simulink model "StateFlow_1"  (R2017b)
settings: Solver=FixedStepDiscrete  StartTime=0.0  StopTime=20000  FixedStep=1  RelTol=1e-3
settings Model: Creator=Administrator  LastModifiedBy=Administrator
settings OptimizationCC: DefaultParameterBehavior=Inlined  UseDivisionForNetSlopeComputation=on  UseFloatMulNetSlope=on  InlineInvariantSignals=on  PassReuseOutputArgsAs=Individual arguments  ZeroExternalMemoryAtStartup=off  ZeroInternalMemoryAtStartup=off  NoFixptDivByZeroProtection=on  EfficientFloat2IntCast=on  LifeSpan=1
settings DebuggingCC: ParameterOverflowMsg=none  ParameterTunabilityLossMsg=error  SFUnexpectedBacktrackingDiag=warning  SFNoUnconditionalDefaultTransitionDiag=warning  SFOutputUsedAsStateInMooreChartDiag=warning
settings HardwareCC: ProdBitPerChar=16  ProdBitPerInt=16  ProdBitPerPointer=32  ProdBitPerSizeT=32  ProdBitPerPtrDiffT=32  ProdLargestAtomicInteger=Integer  ProdLargestAtomicFloat=None  ProdWordSize=16  ProdLongLongMode=on  ProdHWDeviceType=Texas Instruments->C2000
settings SFSimCC: MATLABDynamicMemAlloc=off
settings RTWCC: SystemTargetFile=ert.tlc  TemplateMakefile=ert_default_tmf  GenerateReport=on  IncludeHyperlinkInReport=on  LaunchReport=on  GenerateTraceInfo=on  GenerateTraceReport=on  GenerateTraceReportSl=on  GenerateTraceReportSf=on  GenerateTraceReportEml=on  GenerateCodeMetricsReport=on
settings CodeAppCC: ForceParamTrailComments=on  IgnoreCustomStorageClasses=off  OperatorAnnotations=on  SimulinkDataObjDesc=on  SFDataObjDesc=on  CustomSymbolStrGlobalVar=rt$N$M  CustomSymbolStrType=$N$M  CustomSymbolStrFcn=$N$M$F  CustomSymbolStrMacro=$N$M  InsertBlockDesc=on
settings ERTTargetCC: TargetLangStandard=C99 (ISO)  GenerateSampleERTMain=on  IncludeMdlTerminateFcn=off  CombineSignalStateStructs=on  SupportAbsoluteTime=off  SupportComplex=off  SupportNonInlinedSFcns=on  InlinedParameterPlacement=NonHierarchical  ERTCustomFileTemplate=example_file_process.tlc  ERTFilePackagingFormat=CompactWithDataFile
settings ConfigComp: DVMaxProcessTime=1000  DVTestSuiteOptimization=CombinedObjectives (Nonlinear Extended)  DVDetectFloatOverflow=off

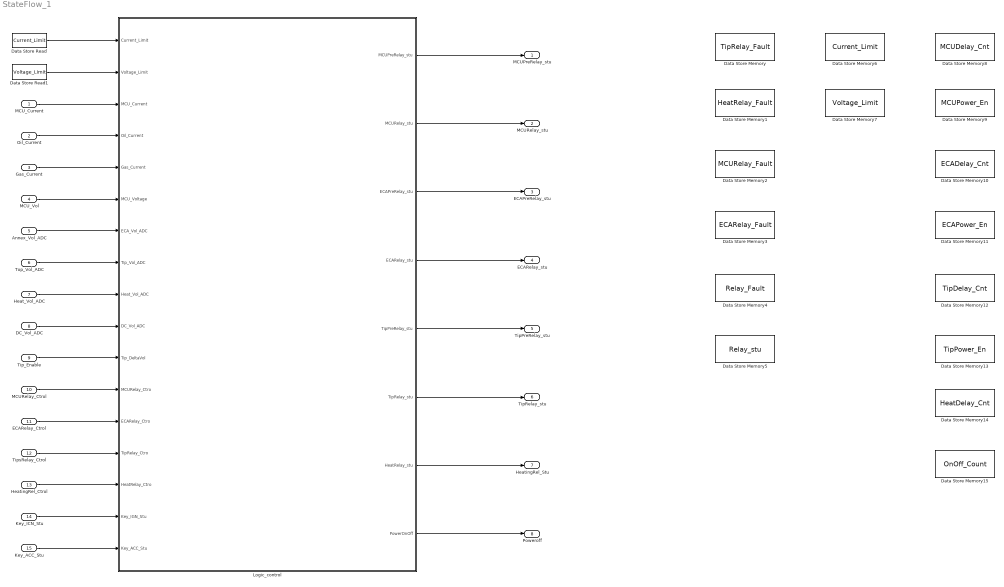
== system StateFlow_1 ==
  MCU_Current : Inport
  Oil_Current : Inport  Port=2
  Gas_Current : Inport  Port=3
  MCU_Vol : Inport  Port=4
  Annex_Vol_ADC : Inport  Port=5
  Top_Vol_ADC : Inport  Port=6
  Heat_Vol_ADC : Inport  Port=7
  DC_Vol_ADC : Inport  Port=8
  Tip_Enable : Inport  Port=9
  MCURelay_Ctrol : Inport  Port=10
  ECARelay_Ctrol : Inport  Port=11
  TipsRelay_Ctrol : Inport  Port=12
  HeatingRel_Ctrol : Inport  Port=13
  Key_ICN_Stu : Inport  Port=14
  Key_ACC_Stu : Inport  Port=15
  Data Store Memory : DataStoreMemory  DataStoreName=TipRelay_Fault  ReadBeforeWriteMsg=warning  WriteAfterWriteMsg=warning  WriteAfterReadMsg=warning  ShowAdditionalParam=off  OutDataTypeStr=uint8
  Data Store Memory1 : DataStoreMemory  DataStoreName=HeatRelay_Fault  ReadBeforeWriteMsg=warning  WriteAfterWriteMsg=warning  WriteAfterReadMsg=warning  ShowAdditionalParam=off  OutDataTypeStr=uint8
  Data Store Memory10 : DataStoreMemory  DataStoreName=ECADelay_Cnt  ReadBeforeWriteMsg=warning  WriteAfterWriteMsg=warning  WriteAfterReadMsg=warning  ShowAdditionalParam=off  OutDataTypeStr=uint16
  Data Store Memory11 : DataStoreMemory  DataStoreName=ECAPower_En  ReadBeforeWriteMsg=warning  WriteAfterWriteMsg=warning  WriteAfterReadMsg=warning  ShowAdditionalParam=off  OutDataTypeStr=uint16
  Data Store Memory12 : DataStoreMemory  DataStoreName=TipDelay_Cnt  ReadBeforeWriteMsg=warning  WriteAfterWriteMsg=warning  WriteAfterReadMsg=warning  ShowAdditionalParam=off  OutDataTypeStr=uint16
  Data Store Memory13 : DataStoreMemory  DataStoreName=TipPower_En  ReadBeforeWriteMsg=warning  WriteAfterWriteMsg=warning  WriteAfterReadMsg=warning  ShowAdditionalParam=off  OutDataTypeStr=uint16
  Data Store Memory14 : DataStoreMemory  DataStoreName=HeatDelay_Cnt  ReadBeforeWriteMsg=warning  WriteAfterWriteMsg=warning  WriteAfterReadMsg=warning  ShowAdditionalParam=off  OutDataTypeStr=uint16
  Data Store Memory15 : DataStoreMemory  DataStoreName=OnOff_Count  ReadBeforeWriteMsg=warning  WriteAfterWriteMsg=warning  WriteAfterReadMsg=warning  ShowAdditionalParam=off  OutDataTypeStr=uint16
  Data Store Memory2 : DataStoreMemory  DataStoreName=MCURelay_Fault  ReadBeforeWriteMsg=warning  WriteAfterWriteMsg=warning  WriteAfterReadMsg=warning  ShowAdditionalParam=off  OutDataTypeStr=uint8
  Data Store Memory3 : DataStoreMemory  DataStoreName=ECARelay_Fault  ReadBeforeWriteMsg=warning  WriteAfterWriteMsg=warning  WriteAfterReadMsg=warning  ShowAdditionalParam=off  OutDataTypeStr=uint8
  Data Store Memory4 : DataStoreMemory  DataStoreName=Relay_Fault  ReadBeforeWriteMsg=warning  WriteAfterWriteMsg=warning  WriteAfterReadMsg=warning  ShowAdditionalParam=off  OutDataTypeStr=uint8
  Data Store Memory5 : DataStoreMemory  DataStoreName=Relay_stu  ReadBeforeWriteMsg=warning  WriteAfterWriteMsg=warning  WriteAfterReadMsg=warning  ShowAdditionalParam=off  OutDataTypeStr=uint8
  Data Store Memory6 : DataStoreMemory  DataStoreName=Current_Limit  ReadBeforeWriteMsg=warning  WriteAfterWriteMsg=warning  WriteAfterReadMsg=warning  InitialValue=15  ShowAdditionalParam=off  OutDataTypeStr=uint16
  Data Store Memory7 : DataStoreMemory  DataStoreName=Voltage_Limit  ReadBeforeWriteMsg=warning  WriteAfterWriteMsg=warning  WriteAfterReadMsg=warning  InitialValue=40  ShowAdditionalParam=off  OutDataTypeStr=uint16
  Data Store Memory8 : DataStoreMemory  DataStoreName=MCUDelay_Cnt  ReadBeforeWriteMsg=warning  WriteAfterWriteMsg=warning  WriteAfterReadMsg=warning  ShowAdditionalParam=off  OutDataTypeStr=uint16
  Data Store Memory9 : DataStoreMemory  DataStoreName=MCUPower_En  ReadBeforeWriteMsg=warning  WriteAfterWriteMsg=warning  WriteAfterReadMsg=warning  ShowAdditionalParam=off  OutDataTypeStr=uint16
  Data Store Read : DataStoreRead  DataStoreName=Current_Limit
  Data Store Read1 : DataStoreRead  DataStoreName=Voltage_Limit
  Logic_control : Subsystem  TreatAsAtomicUnit=on
  MCUPreRelay_stu : Outport
  MCURelay_stu : Outport  Port=2
  ECAPreRelay_stu : Outport  Port=3
  ECARelay_stu : Outport  Port=4
  TipPreRelay_stu : Outport  Port=5
  TipRelay_stu : Outport  Port=6
  HeatingRel_Stu : Outport  Port=7
  Poweroff : Outport  Port=8
  wires:
  Data Store Read/1 -> Logic_control/1(Current_Limit)
  Data Store Read1/1 -> Logic_control/2(Voltage_Limit)
  MCU_Current/1 -> Logic_control/3(MCU_Current)
  Oil_Current/1 -> Logic_control/4(Oil_Current)
  Gas_Current/1 -> Logic_control/5(Gas_Current)
  MCU_Vol/1 -> Logic_control/6(MCU_Voltage)
  MCURelay_Ctrol/1 -> Logic_control/12(MCURelay_Ctro)
  ECARelay_Ctrol/1 -> Logic_control/13(ECARelay_Ctro)
  TipsRelay_Ctrol/1 -> Logic_control/14(TipRelay_Ctro)
  HeatingRel_Ctrol/1 -> Logic_control/15(HeatRelay_Ctro)
  Key_ICN_Stu/1 -> Logic_control/16(Key_IGN_Stu)
  Key_ACC_Stu/1 -> Logic_control/17(Key_ACC_Stu)
  Logic_control/1(MCUPreRelay_stu) -> MCUPreRelay_stu/1
  Logic_control/2(MCURelay_stu) -> MCURelay_stu/1
  Logic_control/3(ECAPreRelay_stu) -> ECAPreRelay_stu/1
  Logic_control/4(ECARelay_stu) -> ECARelay_stu/1
  Logic_control/5(TipPreRelay_stu) -> TipPreRelay_stu/1
  Logic_control/6(TipRelay_stu) -> TipRelay_stu/1
  Logic_control/7(HeatRelay_stu) -> HeatingRel_Stu/1
  Logic_control/8(PowerOnOff) -> Poweroff/1
  Annex_Vol_ADC/1 -> Logic_control/7(ECA_Vol_ADC)
  Top_Vol_ADC/1 -> Logic_control/8(Tip_Vol_ADC)
  Heat_Vol_ADC/1 -> Logic_control/9(Heat_Vol_ADC)
  DC_Vol_ADC/1 -> Logic_control/10(DC_Vol_ADC)
  Tip_Enable/1 -> Logic_control/11(Tip_DeltaVol)

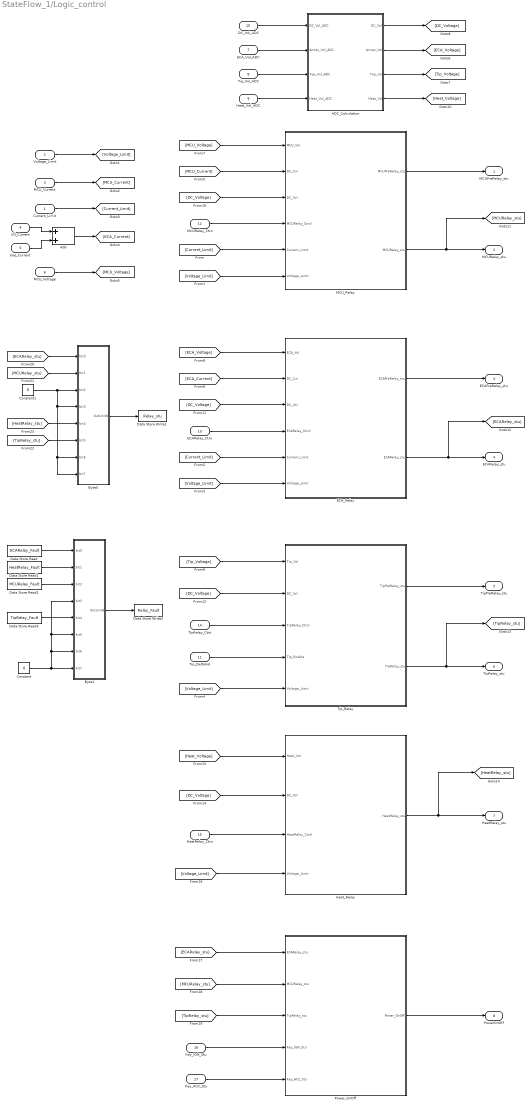
== system StateFlow_1/Logic_control ==
  Current_Limit : Inport
  Voltage_Limit : Inport  Port=2
  MCU_Current : Inport  Port=3
  Oil_Current : Inport  Port=4
  Gas_Current : Inport  Port=5
  MCU_Voltage : Inport  Port=6
  ECA_Vol_ADC : Inport  Port=7
  Tip_Vol_ADC : Inport  Port=8
  Heat_Vol_ADC : Inport  Port=9
  DC_Vol_ADC : Inport  Port=10
  Tip_DeltaVol : Inport  Port=11
  MCURelay_Ctro : Inport  Port=12
  ECARelay_Ctro : Inport  Port=13
  TipRelay_Ctro : Inport  Port=14
  HeatRelay_Ctro : Inport  Port=15
  Key_IGN_Stu : Inport  Port=16
  Key_ACC_Stu : Inport  Port=17
  ADC_Calculation : Subsystem
  Add : Sum
  Byte0 : Subsystem
  Byte1 : Subsystem
  Constant : Constant  Value=0  OutDataTypeStr=uint8
  Constant1 : Constant  Value=0  OutDataTypeStr=uint8
  Data Store Read : DataStoreRead  DataStoreName=ECARelay_Fault
  Data Store Read1 : DataStoreRead  DataStoreName=HeatRelay_Fault
  Data Store Read2 : DataStoreRead  DataStoreName=MCURelay_Fault
  Data Store Read3 : DataStoreRead  DataStoreName=TipRelay_Fault
  Data Store Write1 : DataStoreWrite  DataStoreName=Relay_stu
  Data Store Write2 : DataStoreWrite  DataStoreName=Relay_Fault
  ECA_Relay : Stateflow chart  TreatAsAtomicUnit=on
  Heat_Relay : Stateflow chart  TreatAsAtomicUnit=on
  MCU_Relay : Stateflow chart  TreatAsAtomicUnit=on
  Power_OnOff : Stateflow chart  TreatAsAtomicUnit=on
  Tip_Relay : Stateflow chart  TreatAsAtomicUnit=on
  MCUPreRelay_stu : Outport
  MCURelay_stu : Outport  Port=2
  ECAPreRelay_stu : Outport  Port=3
  ECARelay_stu : Outport  Port=4
  TipPreRelay_stu : Outport  Port=5
  TipRelay_stu : Outport  Port=6
  HeatRelay_stu : Outport  Port=7
  PowerOnOff : Outport  Port=8
  wires:
  [ECARelay_stu] -> Byte0/1(bit0)
  MCU_Relay/2(MCURelay_stu) -> [MCURelay_stu], MCURelay_stu/1
  MCU_Relay/1(MCUPreRelay_stu) -> MCUPreRelay_stu/1
  [MCURelay_stu] -> Power_OnOff/2(MCURelay_stu)
  TipRelay_Ctro/1 -> Tip_Relay/3(TipRelay_Ctrol)
  Key_IGN_Stu/1 -> Power_OnOff/4(Key_IGN_Stu)
  Tip_DeltaVol/1 -> Tip_Relay/4(Tip_Enable)
  [Voltage_Limit] -> ECA_Relay/6(Voltage_Limit)
  Tip_Relay/1(TipPreRelay_stu) -> TipPreRelay_stu/1
  Tip_Relay/2(TipRelay_stu) -> [TipRelay_stu], TipRelay_stu/1
  [MCU_Voltage] -> MCU_Relay/1(MCU_Vol)
  Heat_Relay/1(HeatRelay_stu) -> [HeatRelay_stu], HeatRelay_stu/1
  Voltage_Limit/1 -> [Voltage_Limit]
  Current_Limit/1 -> [Current_Limit]
  Data Store Read/1 -> Byte1/1(bit0)
  [DC_Voltage] -> Heat_Relay/2(DC_Vol)
  ECA_Relay/1(ECAPreRelay_stu) -> ECAPreRelay_stu/1
  MCU_Current/1 -> [MCU_Current]
  [Voltage_Limit] -> Tip_Relay/5(Voltage_Limit)
  [Heat_Voltage] -> Heat_Relay/1(Heat_Vol)
  MCU_Voltage/1 -> [MCU_Voltage]
  Data Store Read3/1 -> Byte1/5(bit4)
  Constant/1 -> Byte1/7(bit6), Byte1/6(bit5), Byte1/4(bit3), Byte1/8(bit7)
  [Voltage_Limit] -> Heat_Relay/4(Voltage_Limit)
  [DC_Voltage] -> ECA_Relay/3(DC_Vol)
  Power_OnOff/1(Power_OnOff) -> PowerOnOff/1
  ECARelay_Ctro/1 -> ECA_Relay/4(ECARelay_Ctrol)
  Add/1 -> [ECA_Current]
  [MCU_Current] -> MCU_Relay/2(DC_Cur)
  [MCURelay_stu] -> Byte0/2(bit1)
  [TipRelay_stu] -> Byte0/6(bit5)
  [ECA_Current] -> ECA_Relay/2(DC_Cur)
  Gas_Current/1 -> Add/2
  HeatRelay_Ctro/1 -> Heat_Relay/3(HeatRelay_Ctrol)
  Byte1/1(OutUnit8) -> Data Store Write2/1
  ECA_Relay/2(ECARelay_stu) -> [ECARelay_stu], ECARelay_stu/1
  Constant1/1 -> Byte0/4(bit3), Byte0/7(bit6), Byte0/8(bit7), Byte0/3(bit2)
  Data Store Read2/1 -> Byte1/3(bit2)
  [DC_Voltage] -> Tip_Relay/2(DC_Vol)
  Oil_Current/1 -> Add/1
  [Current_Limit] -> ECA_Relay/5(Current_Limit)
  Key_ACC_Stu/1 -> Power_OnOff/5(Key_ACC_Stu)
  [Tip_Voltage] -> Tip_Relay/1(Tip_Vol)
  Byte0/1(OutUnit8) -> Data Store Write1/1
  [HeatRelay_stu] -> Byte0/5(bit4)
  [ECARelay_stu] -> Power_OnOff/1(ECARelay_stu)
  MCURelay_Ctro/1 -> MCU_Relay/4(MCURelay_Ctrol)
  [Voltage_Limit] -> MCU_Relay/6(Voltage_Limit)
  Data Store Read1/1 -> Byte1/2(bit1)
  [TipRelay_stu] -> Power_OnOff/3(TipRelay_stu)
  [DC_Voltage] -> MCU_Relay/3(DC_Vol)
  [Current_Limit] -> MCU_Relay/5(Current_Limit)
  [ECA_Voltage] -> ECA_Relay/1(ECA_Vol)
  DC_Vol_ADC/1 -> ADC_Calculation/1(DC_Vol_ADC)
  ECA_Vol_ADC/1 -> ADC_Calculation/2(Annex_Vol_ADC)
  Tip_Vol_ADC/1 -> ADC_Calculation/3(Top_Vol_ADC)
  Heat_Vol_ADC/1 -> ADC_Calculation/4(Heat_Vol_ADC)
  ADC_Calculation/1(DC_Vol) -> [DC_Voltage]
  ADC_Calculation/2(Annex_Vol) -> [ECA_Voltage]
  ADC_Calculation/3(Top_Vol) -> [Tip_Voltage]
  ADC_Calculation/4(Heat_Vol) -> [Heat_Voltage]

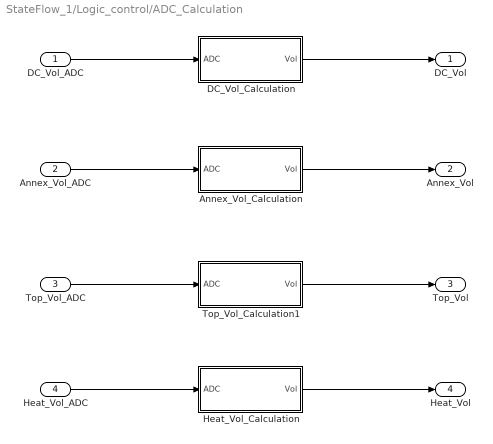
== system StateFlow_1/Logic_control/ADC_Calculation ==
  DC_Vol_ADC : Inport
  Annex_Vol_ADC : Inport  Port=2
  Top_Vol_ADC : Inport  Port=3
  Heat_Vol_ADC : Inport  Port=4
  Annex_Vol_Calculation : Subsystem
  DC_Vol_Calculation : Subsystem
  Heat_Vol_Calculation : Subsystem
  Top_Vol_Calculation1 : Subsystem
  DC_Vol : Outport
  Annex_Vol : Outport  Port=2
  Top_Vol : Outport  Port=3
  Heat_Vol : Outport  Port=4
  wires:
  DC_Vol_ADC/1 -> DC_Vol_Calculation/1(ADC)
  DC_Vol_Calculation/1(Vol) -> DC_Vol/1
  Annex_Vol_ADC/1 -> Annex_Vol_Calculation/1(ADC)
  Annex_Vol_Calculation/1(Vol) -> Annex_Vol/1
  Top_Vol_ADC/1 -> Top_Vol_Calculation1/1(ADC)
  Top_Vol_Calculation1/1(Vol) -> Top_Vol/1
  Heat_Vol_ADC/1 -> Heat_Vol_Calculation/1(ADC)
  Heat_Vol_Calculation/1(Vol) -> Heat_Vol/1

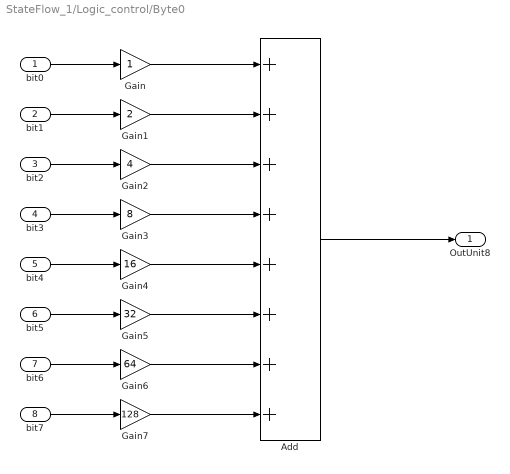
== system StateFlow_1/Logic_control/Byte0 ==
  bit0 : Inport  OutDataTypeStr=uint8
  bit1 : Inport  Port=2
  bit2 : Inport  Port=3
  bit3 : Inport  Port=4
  bit4 : Inport  Port=5
  bit5 : Inport  Port=6
  bit6 : Inport  Port=7
  bit7 : Inport  Port=8
  Add : Sum  Inputs=++++++++  OutDataTypeStr=uint8
  Gain : Gain
  Gain1 : Gain  Gain=2
  Gain2 : Gain  Gain=4
  Gain3 : Gain  Gain=8
  Gain4 : Gain  Gain=16
  Gain5 : Gain  Gain=32
  Gain6 : Gain  Gain=64
  Gain7 : Gain  Gain=128
  OutUnit8 : Outport
  wires:
  bit0/1 -> Gain/1
  Gain/1 -> Add/1
  bit1/1 -> Gain1/1
  Gain1/1 -> Add/2
  bit2/1 -> Gain2/1
  Gain2/1 -> Add/3
  bit3/1 -> Gain3/1
  Gain3/1 -> Add/4
  bit4/1 -> Gain4/1
  Gain4/1 -> Add/5
  bit5/1 -> Gain5/1
  Gain5/1 -> Add/6
  bit6/1 -> Gain6/1
  Gain6/1 -> Add/7
  bit7/1 -> Gain7/1
  Gain7/1 -> Add/8
  Add/1 -> OutUnit8/1

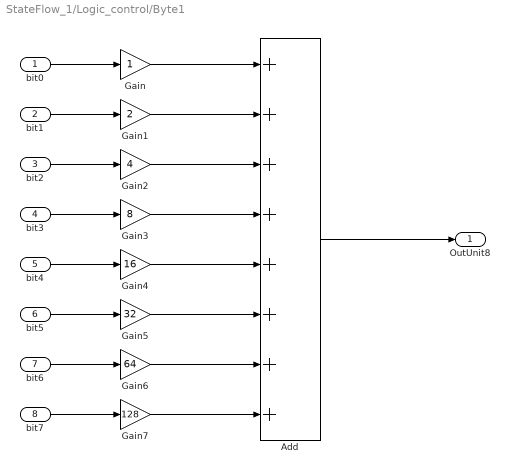
== system StateFlow_1/Logic_control/Byte1 ==
  bit0 : Inport  OutDataTypeStr=uint8
  bit1 : Inport  Port=2  OutDataTypeStr=uint8
  bit2 : Inport  Port=3
  bit3 : Inport  Port=4
  bit4 : Inport  Port=5
  bit5 : Inport  Port=6
  bit6 : Inport  Port=7
  bit7 : Inport  Port=8
  Add : Sum  Inputs=++++++++  OutDataTypeStr=uint8
  Gain : Gain
  Gain1 : Gain  Gain=2
  Gain2 : Gain  Gain=4
  Gain3 : Gain  Gain=8
  Gain4 : Gain  Gain=16
  Gain5 : Gain  Gain=32
  Gain6 : Gain  Gain=64
  Gain7 : Gain  Gain=128
  OutUnit8 : Outport
  wires:
  bit0/1 -> Gain/1
  Gain/1 -> Add/1
  bit1/1 -> Gain1/1
  Gain1/1 -> Add/2
  bit2/1 -> Gain2/1
  Gain2/1 -> Add/3
  bit3/1 -> Gain3/1
  Gain3/1 -> Add/4
  bit4/1 -> Gain4/1
  Gain4/1 -> Add/5
  bit5/1 -> Gain5/1
  Gain5/1 -> Add/6
  bit6/1 -> Gain6/1
  Gain6/1 -> Add/7
  bit7/1 -> Gain7/1
  Gain7/1 -> Add/8
  Add/1 -> OutUnit8/1

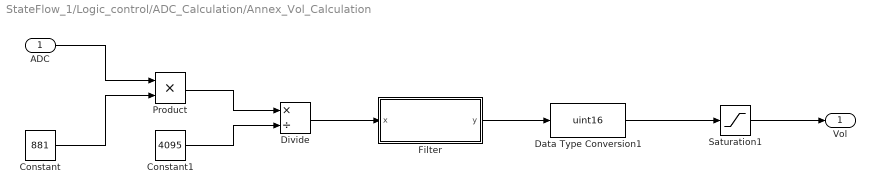
== system StateFlow_1/Logic_control/ADC_Calculation/Annex_Vol_Calculation ==
  ADC : Inport
  Constant : Constant  Value=881
  Constant1 : Constant  Value=4095
  Data Type Conversion1 : DataTypeConversion  OutDataTypeStr=uint16
  Divide : Product  Inputs=*/
  Filter : Subsystem
  Product : Product
  Saturation1 : Saturate  UpperLimit=inf  LowerLimit=0
  Vol : Outport
  wires:
  Filter/1(y) -> Data Type Conversion1/1
  Data Type Conversion1/1 -> Saturation1/1
  Constant/1 -> Product/2
  Constant1/1 -> Divide/2
  Product/1 -> Divide/1
  Divide/1 -> Filter/1(x)
  ADC/1 -> Product/1
  Saturation1/1 -> Vol/1

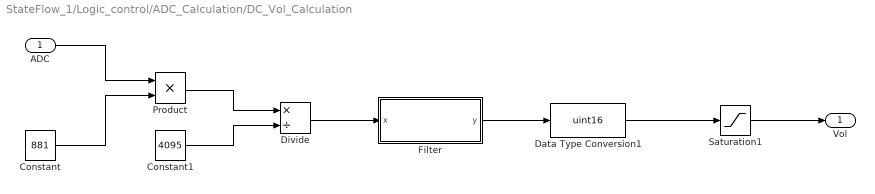
== system StateFlow_1/Logic_control/ADC_Calculation/DC_Vol_Calculation ==
  ADC : Inport
  Constant : Constant  Value=881
  Constant1 : Constant  Value=4095
  Data Type Conversion1 : DataTypeConversion  OutDataTypeStr=uint16
  Divide : Product  Inputs=*/
  Filter : Subsystem
  Product : Product
  Saturation1 : Saturate  UpperLimit=inf  LowerLimit=0
  Vol : Outport
  wires:
  ADC/1 -> Product/1
  Constant/1 -> Product/2
  Product/1 -> Divide/1
  Constant1/1 -> Divide/2
  Divide/1 -> Filter/1(x)
  Filter/1(y) -> Data Type Conversion1/1
  Data Type Conversion1/1 -> Saturation1/1
  Saturation1/1 -> Vol/1

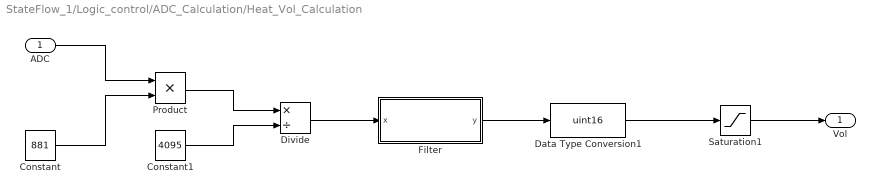
== system StateFlow_1/Logic_control/ADC_Calculation/Heat_Vol_Calculation ==
  ADC : Inport
  Constant : Constant  Value=881
  Constant1 : Constant  Value=4095
  Data Type Conversion1 : DataTypeConversion  OutDataTypeStr=uint16
  Divide : Product  Inputs=*/
  Filter : Subsystem
  Product : Product
  Saturation1 : Saturate  UpperLimit=inf  LowerLimit=0
  Vol : Outport
  wires:
  Divide/1 -> Filter/1(x)
  Filter/1(y) -> Data Type Conversion1/1
  Saturation1/1 -> Vol/1
  Data Type Conversion1/1 -> Saturation1/1
  Constant/1 -> Product/2
  ADC/1 -> Product/1
  Constant1/1 -> Divide/2
  Product/1 -> Divide/1

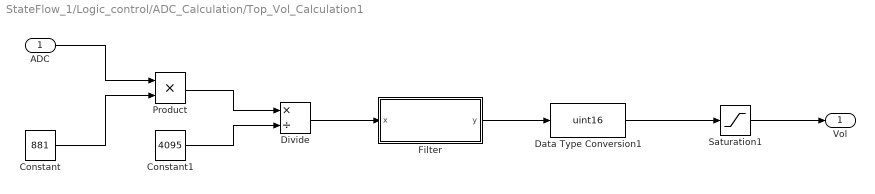
== system StateFlow_1/Logic_control/ADC_Calculation/Top_Vol_Calculation1 ==
  ADC : Inport
  Constant : Constant  Value=881
  Constant1 : Constant  Value=4095
  Data Type Conversion1 : DataTypeConversion  OutDataTypeStr=uint16
  Divide : Product  Inputs=*/
  Filter : Subsystem
  Product : Product
  Saturation1 : Saturate  UpperLimit=inf  LowerLimit=0
  Vol : Outport
  wires:
  Divide/1 -> Filter/1(x)
  Filter/1(y) -> Data Type Conversion1/1
  Saturation1/1 -> Vol/1
  Data Type Conversion1/1 -> Saturation1/1
  Constant/1 -> Product/2
  ADC/1 -> Product/1
  Constant1/1 -> Divide/2
  Product/1 -> Divide/1

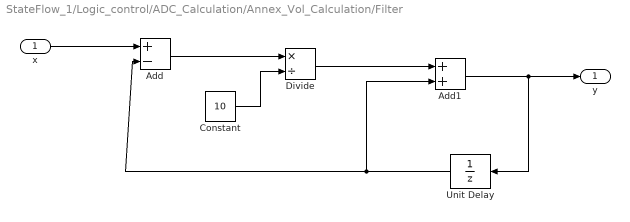
== system StateFlow_1/Logic_control/ADC_Calculation/Annex_Vol_Calculation/Filter ==
  x : Inport
  Add : Sum  Inputs=+-
  Add1 : Sum
  Constant : Constant  Value=10
  Divide : Product  Inputs=*/
  Unit Delay : UnitDelay  SampleTime=-1
  y : Outport
  wires:
  x/1 -> Add/1
  Add/1 -> Divide/1
  Divide/1 -> Add1/1
  Add1/1 -> Unit Delay/1, y/1
  Constant/1 -> Divide/2
  Unit Delay/1 -> Add1/2, Add/2

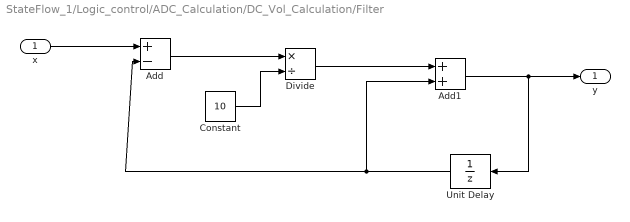
== system StateFlow_1/Logic_control/ADC_Calculation/DC_Vol_Calculation/Filter ==
  x : Inport
  Add : Sum  Inputs=+-
  Add1 : Sum
  Constant : Constant  Value=10
  Divide : Product  Inputs=*/
  Unit Delay : UnitDelay  SampleTime=-1
  y : Outport
  wires:
  x/1 -> Add/1
  Add/1 -> Divide/1
  Divide/1 -> Add1/1
  Add1/1 -> Unit Delay/1, y/1
  Constant/1 -> Divide/2
  Unit Delay/1 -> Add1/2, Add/2

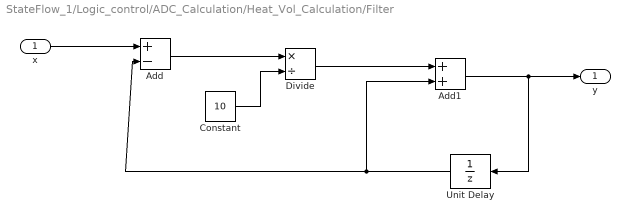
== system StateFlow_1/Logic_control/ADC_Calculation/Heat_Vol_Calculation/Filter ==
  x : Inport
  Add : Sum  Inputs=+-
  Add1 : Sum
  Constant : Constant  Value=10
  Divide : Product  Inputs=*/
  Unit Delay : UnitDelay  SampleTime=-1
  y : Outport
  wires:
  x/1 -> Add/1
  Add/1 -> Divide/1
  Divide/1 -> Add1/1
  Add1/1 -> Unit Delay/1, y/1
  Constant/1 -> Divide/2
  Unit Delay/1 -> Add1/2, Add/2

== system StateFlow_1/Logic_control/ADC_Calculation/Top_Vol_Calculation1/Filter ==
  x : Inport
  Add : Sum  Inputs=+-
  Add1 : Sum
  Constant : Constant  Value=10
  Divide : Product  Inputs=*/
  Unit Delay : UnitDelay  SampleTime=-1
  y : Outport
  wires:
  x/1 -> Add/1
  Add/1 -> Divide/1
  Divide/1 -> Add1/1
  Add1/1 -> Unit Delay/1, y/1
  Constant/1 -> Divide/2
  Unit Delay/1 -> Add1/2, Add/2

== stateflow chart StateFlow_1/Logic_control/ECA_Relay ==
  (default) -> (junction 95)
  (junction 97) -> (junction 109) [order 2] : [DC_Cur<Current_Limit]
  (junction 95) -> (junction 97) [order 1] : [ECARelay_Ctrol==0]
      | {ECADelay_Cnt=0;}
  (junction 95) -> (junction 98) [order 2] : [ECARelay_Ctrol==1]
  (junction 98) -> (junction 105) [order 2] : [ECAPower_En == 1]
  (junction 109) -> (junction 111) : {ECARelay_stu = 0;
      | ECAPreRelay_stu=0;}
  (junction 97) -> (junction 110) [order 1] : [DC_Cur>=Current_Limit]
  (junction 95) -> (junction 99) [order 3] : [ECARelay_Fault==1]
  (junction 98) -> (junction 103) [order 1] : [ECAPower_En == 0]
  (junction 105) -> (junction 119) : [(ECARelay_Fault ==0)]
      | {ECAPreRelay_stu=1;
      | ECADelay_Cnt = ECADelay_Cnt + 1;}
  (junction 111) -> (junction 110)
  (junction 110) -> (junction 99)
  (junction 103) -> (junction 99) : [(ECAPreRelay_stu==0)&&(ECARelay_stu==0)]
      | {ECAPower_En =1;}
  (junction 99) -> (junction 118)
  (junction 119) -> (junction 118) [order 2] : [ECADelay_Cnt<=1000]
  (junction 118) -> (junction 123)
  (junction 119) -> (junction 124) [order 1] : [ECADelay_Cnt>1000]
  (junction 124) -> (junction 123) [order 1] : [abs(DC_Vol-ECA_Vol)>=Voltage_Limit]
      | {ECARelay_Fault=1;
      | ECADelay_Cnt=0;
      | ECAPower_En=0;
      | ECAPreRelay_stu=0;}
  (junction 123) -> (junction 131)
  (junction 124) -> (junction 132) [order 2] : [abs(DC_Vol-ECA_Vol)<Voltage_Limit]
  (junction 132) -> (junction 131) [order 1] : [ECADelay_Cnt<1500]
  (junction 131) -> (junction 135)
  (junction 132) -> (junction 136) [order 2] : [ECADelay_Cnt>1500]
      | {ECARelay_stu=1;}
  (junction 136) -> (junction 135) [order 2] : [ECADelay_Cnt<2000]
  (junction 135) -> (junction 138)
  (junction 136) -> (junction 139) [order 1] : [ECADelay_Cnt>=2000]
      | {ECAPreRelay_stu=0;
      | ECADelay_Cnt=0;
      | ECAPower_En = 0;}
  (junction 139) -> (junction 138)
  (junction 138) -> (junction 146)
  data: ECA_Vol input; DC_Cur input; DC_Vol input; ECARelay_Ctrol input; Current_Limit input; Voltage_Limit input; ECAPreRelay_stu output; ECARelay_stu output uint8; ECADelay_Cnt data_store_memory; ECAPower_En data_store_memory; ECARelay_Fault data_store_memory

== stateflow chart StateFlow_1/Logic_control/Tip_Relay ==
  (default) -> (junction 98)
  (junction 98) -> (junction 96) : {TipControl_stu=TipRelay_Ctrol;}
  (junction 96) -> (junction 95) [order 2]
  (junction 96) -> (junction 95) [order 1] : [Tip_Enable==0]
      | {TipControl_stu=0;}
  (junction 95) -> (junction 121)
  (junction 108) -> (junction 113) [order 2] : [abs(Tip_Vol-DC_Vol)>Voltage_Limit]
  (junction 121) -> (junction 108) [order 1] : [TipControl_stu==0]
      | {TipDelay_Cnt=0;}
  (junction 121) -> (junction 112) [order 2] : [TipControl_stu==1]
  (junction 112) -> (junction 111) [order 2] : [TipPower_En == 1]
  (junction 113) -> (junction 97) : {TipDelay_Cnt = TipDelay_Cnt + 1;}
  (junction 108) -> (junction 101) [order 1] : [abs(Tip_Vol-DC_Vol)<=Voltage_Limit]
  (junction 121) -> (junction 99) [order 3] : [TipRelay_Fault == 1]
  (junction 112) -> (junction 120) [order 1] : [TipPower_En == 0]
  (junction 111) -> (junction 128) : [(TipRelay_Fault ==0)]
      | {TipPreRelay_stu=1;
      | TipDelay_Cnt = TipDelay_Cnt + 1;}
  (junction 120) -> (junction 99) : [(TipPreRelay_stu==0)&&(TipRelay_stu==0)]
      | {TipPower_En =1;}
  (junction 99) -> (junction 103)
  (junction 97) -> (junction 101) [order 1] : [TipDelay_Cnt>=2000]
  (junction 101) -> (junction 103) : {TipRelay_stu=0;
      | TipPreRelay_stu=0;
      | TipDelay_Cnt=0;}
  (junction 103) -> (junction 104)
  (junction 97) -> (junction 126) [order 2] : [TipDelay_Cnt<2000]
  (junction 126) -> (junction 104)
  (junction 128) -> (junction 104) [order 2] : [TipDelay_Cnt<=1000]
  (junction 128) -> (junction 110) [order 1] : [TipDelay_Cnt>1000]
  (junction 104) -> (junction 114)
  (junction 110) -> (junction 114) [order 1] : [abs(DC_Vol-Tip_Vol)>=Voltage_Limit]
      | {TipRelay_Fault=1;
      | TipDelay_Cnt=0;
      | TipPower_En=0;
      | TipPreRelay_stu=0;}
  (junction 114) -> (junction 107)
  (junction 110) -> (junction 105) [order 2] : [abs(DC_Vol-Tip_Vol)<Voltage_Limit]
  (junction 105) -> (junction 107) [order 1] : [TipDelay_Cnt<1500]
  (junction 107) -> (junction 127)
  (junction 105) -> (junction 119) [order 2] : [TipDelay_Cnt>1500]
      | {TipRelay_stu=1;}
  (junction 119) -> (junction 127) [order 2] : [TipDelay_Cnt<2000]
  (junction 127) -> (junction 125)
  (junction 119) -> (junction 123) [order 1] : [TipDelay_Cnt>=2000]
      | {TipPreRelay_stu=0;
      | TipDelay_Cnt=0;
      | TipPower_En = 0;
      | }
  (junction 123) -> (junction 125)
  (junction 125) -> (junction 124)
  data: Tip_Vol input; DC_Vol input; TipPreRelay_stu output; TipRelay_stu output; TipControl_stu local; TipDelay_Cnt data_store_memory; TipPower_En data_store_memory; TipRelay_Fault data_store_memory; TipRelay_Ctrol input; Tip_Enable input; Voltage_Limit input

== stateflow chart StateFlow_1/Logic_control/MCU_Relay ==
  (default) -> (junction 14)
  (junction 25) -> (junction 29) [order 2] : [DC_Cur<Current_Limit]
  (junction 14) -> (junction 25) [order 1] : [MCURelay_Ctrol==0]
      | {MCUDelay_Cnt  = 0;}
  (junction 14) -> (junction 15) [order 2] : [MCURelay_Ctrol==1]
  (junction 15) -> (junction 27) [order 2] : [MCUPower_En == 1]
  (junction 29) -> (junction 39) : {MCURelay_stu= 0;
      | MCUPreRelay_stu=0;}
  (junction 25) -> (junction 38) [order 1] : [DC_Cur>=Current_Limit]
  (junction 14) -> (junction 31) [order 3] : [MCURelay_Fault == 1]
  (junction 15) -> (junction 36) [order 1] : [MCUPower_En == 0]
  (junction 27) -> (junction 61) : [(MCURelay_Fault ==0)]{MCUPreRelay_stu=1;
      | MCUDelay_Cnt = MCUDelay_Cnt + 1;}
  (junction 39) -> (junction 38)
  (junction 38) -> (junction 31)
  (junction 36) -> (junction 31) [order 1] : [(MCUPreRelay_stu==0)&&(MCURelay_stu==0)&&(MCU_Vol<Voltage_Limit)]
      | {MCUPower_En =1;}
  (junction 36) -> (junction 54) [order 3] : {MCURelay_stu==1}
  (junction 31) -> (junction 54)
  (junction 36) -> (junction 55) [order 2] : [(MCUPreRelay_stu==0)&&(MCURelay_stu==0)&&(MCU_Vol>Voltage_Limit)]
      | {MCURelay_Fault = 1;
      | MCUPower_En=0;}
  (junction 55) -> (junction 54)
  (junction 54) -> (junction 60)
  (junction 61) -> (junction 60) [order 1] : [MCUDelay_Cnt<=1000]
  (junction 60) -> (junction 65)
  (junction 61) -> (junction 66) [order 2] : [MCUDelay_Cnt>1500]{MCURelay_stu=1;}
  (junction 66) -> (junction 65) [order 1] : [MCUDelay_Cnt<1500]
  (junction 65) -> (junction 69)
  (junction 66) -> (junction 70) [order 2] : [MCUDelay_Cnt>1500]{MCURelay_stu=1;}
  (junction 70) -> (junction 69) [order 2] : [MCUDelay_Cnt<2000]
  (junction 70) -> (junction 76) [order 1] : [MCUDelay_Cnt>=2000]
      | {MCUPreRelay_stu=0;
      | MCUDelay_Cnt=0;
      | MCUPower_En = 0;}
  (junction 69) -> (junction 75)
  (junction 76) -> (junction 75)
  (junction 75) -> (junction 81)
  data: MCU_Vol input; DC_Cur input; MCUPower_En data_store_memory; MCURelay_Fault data_store_memory; MCUDelay_Cnt data_store_memory; MCUPreRelay_stu output; MCURelay_stu output; DC_Vol input; MCURelay_Ctrol input; Current_Limit input; Voltage_Limit input

== stateflow chart StateFlow_1/Logic_control/Heat_Relay ==
  (default) -> (junction 126)
  (junction 126) -> (junction 96) [order 1] : [HeatRelay_Ctrol==0]
      | {HeatDelay_Cnt=0;}
  (junction 126) -> (junction 127) [order 2] : [HeatRelay_Ctrol==1]
  (junction 127) -> (junction 113) [order 2] : [HeatRelay_Fault==0]
  (junction 96) -> (junction 121) : {HeatRelay_stu=0;}
  (junction 126) -> (junction 118) [order 3]
  (junction 127) -> (junction 120) [order 1] : [HeatRelay_Fault==1]
  (junction 113) -> (junction 98) : {HeatRelay_stu=1;
      | HeatDelay_Cnt = HeatDelay_Cnt + 1;}
  (junction 121) -> (junction 118)
  (junction 120) -> (junction 118) : {HeatRelay_stu=0;}
  (junction 118) -> (junction 115)
  (junction 98) -> (junction 116)
  (junction 116) -> (junction 115) [order 1] : [HeatDelay_Cnt<1000]
  (junction 115) -> (junction 109)
  (junction 116) -> (junction 114) [order 2] : [HeatDelay_Cnt>1000]
  (junction 114) -> (junction 109) [order 1] : [abs(DC_Vol-Heat_Vol)<Voltage_Limit]
      | {HeatDelay_Cnt=0;}
  (junction 109) -> (junction 112)
  (junction 114) -> (junction 111) [order 2] : [abs(DC_Vol-Heat_Vol)>=Voltage_Limit]
      | {HeatRelay_Fault=1;
      | HeatDelay_Cnt=0;}
  (junction 111) -> (junction 112)
  data: Heat_Vol input; DC_Vol input; HeatRelay_Ctrol input; Voltage_Limit input; HeatRelay_stu output; HeatDelay_Cnt data_store_memory; HeatRelay_Fault data_store_memory

== stateflow chart StateFlow_1/Logic_control/Power_OnOff ==
  (default) -> (junction 109)
  (junction 109) -> (junction 110) [order 2] : [(Key_IGN_Stu==0)||(Key_ACC_Stu==0)]
  (junction 110) -> (junction 108)
  (junction 109) -> (junction 106) [order 1] : [(Key_IGN_Stu==1)&&(Key_ACC_Stu==1)]
      | {Power_OnOff=1;
      | OnOff_Count = 0;}
  (junction 108) -> (junction 106) [order 1] : [(ECARelay_stu==1)||(MCURelay_stu==1)||(TipRelay_stu==1)]
  (junction 106) -> (junction 101)
  (junction 108) -> (junction 103) [order 2] : [(ECARelay_stu==0)&&(MCURelay_stu==0)&&(TipRelay_stu==0)]
      | {OnOff_Count = OnOff_Count + 1;}
  (junction 103) -> (junction 101) [order 1] : [OnOff_Count<5000]
  (junction 103) -> (junction 105) [order 2] : [OnOff_Count>=5000]
  (junction 101) -> (junction 100)
  (junction 105) -> (junction 100) : {Power_OnOff=0;
      | OnOff_Count=0;}
  data: ECARelay_stu input uint8; MCURelay_stu input; TipRelay_stu input; Key_IGN_Stu input; Key_ACC_Stu input; Power_OnOff output; OnOff_Count data_store_memory
